simulink model "penddemo"  (R2024a)
settings: Solver=FixedStepAuto  StartTime=0  StopTime=50  FixedStep=0.02  MaxStep=0.02  RelTol=1e-3  AbsTol=1e-6
libraries: slpidlib x1
CloseFcn:
  | set(groot,'ShowHiddenHandles','on');
  | c = get(groot,'Children');
  | close(c);
  | clear c;
  | set(groot,'ShowHiddenHandles','off');
Description:
  | Inverted Pendulum with Animation
  | 
  | This example shows how to model an inverted pendulum.  The animation is created using MATLAB(R) Handle Graphics(R).  The animation block is a masked
  | S-function.  For more information, use the context menu to look under the Animation block's mask
  | and open the S-function for editing.
settings Model: Creator=The MathWorks, Inc.  LastModifiedBy=alexivanov
settings SolverCC: AutoScaleAbsTol=off  AlgebraicLoopSolver=TrustRegion
settings DataIOCC: ExternalInput=[]  InitialState=[]  SaveFormat=Array  SaveOutput=off  SaveTime=off
settings OptimizationCC: BlockReduction=off  BooleanDataType=off  ReuseModelBlockBuffer=off  ExpressionDepthLimit=2147483647  InitFltsAndDblsToZero=on  LifeSpan=inf
settings DebuggingCC: SaveWithParameterizedLinksMsg=none  UnderspecifiedInitializationDetection=Classic  MergeDetectMultiDrivingBlocksExec=none  SignalResolutionControl=TryResolveAllWithWarning  MultiTaskDSMMsg=warning  MultiTaskCondExecSysMsg=none  SigSpecEnsureSampleTimeMsg=none  FcnCallInpInsideContextMsg=warning  UnconnectedInputMsg=warning  UnconnectedOutputMsg=warning  UnconnectedLineMsg=warning  StateNameClashWarn=warning  SubsystemReferenceDiagnosticForUnitTest=warning  SFUnexpectedBacktrackingDiag=warning  SFNoUnconditionalDefaultTransitionDiag=warning  SFExecutionAtInitializationDiag=none  ArithmeticOperatorsInVariantConditions=warning
settings HardwareCC: ProdBitPerPointer=32  ProdBitPerSizeT=32  ProdBitPerPtrDiffT=32  ProdLargestAtomicFloat=None  ProdIntDivRoundTo=Undefined  ProdEndianess=Unspecified  ProdWordSize=32  ProdHWDeviceType=32-bit Generic  TargetUnknown=on
settings ModelReferenceCC: EnableRefExpFcnMdlSchedulingChecks=on  PropagateSignalLabelsOutOfModel=off
settings SFSimCC: SimUseLocalCustomCode=off  CustomCodeUndefinedFunction=UseInterfaceOnly
settings RTWCC: RTWUseLocalCustomCode=off  GPUComputeCapability=3.5
settings CodeAppCC: StateflowObjectComments=on
settings GRTTargetCC: TargetFcnLib=ansi_tfl_tmw.mat  TargetLangStandard=C89/C90 (ANSI)  CombineOutputUpdateFcns=off  GRTInterface=on
settings ConfigComp: CovMetricSettings=dw  CovSaveCumulativeToWorkspaceVar=on  CovSaveSingleToWorkspaceVar=on  CovExternalEMLEnable=off

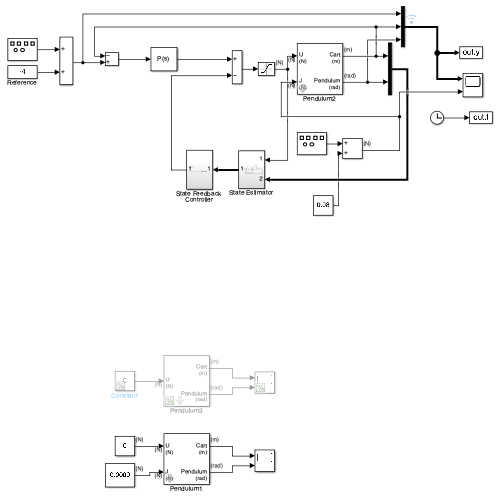
[thumbnail: Simulink's stored preview of the top-level diagram]
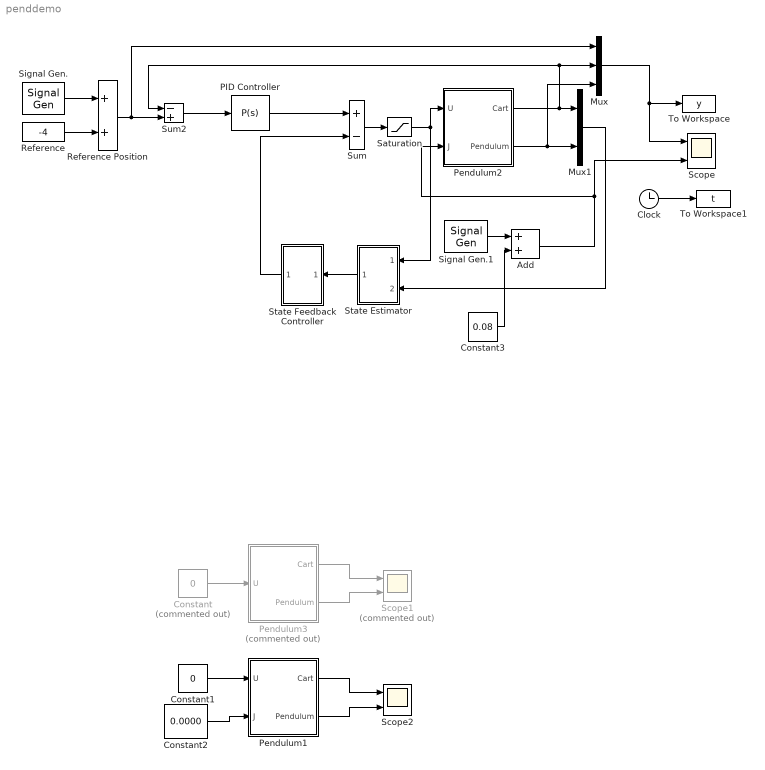
== system penddemo ==
  Add : Sum
  Clock : Clock
  Constant : Constant  Commented=on  Value=0
  Constant1 : Constant  Value=0
  Constant2 : Constant  Value=0.0000
  Constant3 : Constant  Value=0.08
  Mux : Mux  Inputs=3
  Mux1 : Mux  Inputs=2
  "PID Controller " : slpidlib/PID Controller  Controller=P  Form=Parallel  TimeDomain=Continuous-time  UseExternalTs=off  SampleTime=-1  IntegratorMethod=Forward Euler  FilterMethod=Forward Euler  ControllerParametersSource=internal  P=-9.4-4  I=-5  UseKiTs=off  D=0  UseExternalDerivativeSource=off  N=100  UseFilter=on  TunerSelectOption=Transfer Function Based (PID Tuner App)  InitialConditionSource=internal  InitialConditionForIntegrator=0  InitialConditionForFilter=0  DifferentiatorICPrevScaledInput=0  ExternalReset=none  TrackingMode=off  Kt=1  LimitOutput=off  SatLimitsSource=internal  UpperSaturationLimit=inf  LowerSaturationLimit=-inf  LinearizeAsGain=on  AntiWindupMode=none  Kb=1  LimitIntegrator=off  UpperIntegratorSaturationLimit=inf  LowerIntegratorSaturationLimit=-inf  POutMin=[]  POutMax=[]  IOutMin=[]  IOutMax=[]  DOutMin=[]  DOutMax=[]  NOutMin=[]  NOutMax=[]  SumOutMin=[]  SumOutMax=[]  SaturationOutMin=[]  SaturationOutMax=[]  PParamMin=[]  PParamMax=[]  IParamMin=[]  IParamMax=[]  DParamMin=[]  DParamMax=[]  NParamMin=[]  NParamMax=[]  KbParamMin=[]  KbParamMax=[]  KtParamMin=[]  KtParamMax=[]  KbOutMin=[]  KbOutMax=[]  KtOutMin=[]  KtOutMax=[]  IntegratorOutMin=[]  IntegratorOutMax=[]  FilterOutMin=[]  FilterOutMax=[]  SumI1OutMin=[]  SumI1OutMax=[]  SumI2OutMin=[]  SumI2OutMax=[]  SumI3OutMin=[]  SumI3OutMax=[]  SumI4OutMin=[]  SumI4OutMax=[]  SumDOutMin=[]  SumDOutMax=[]  DifferentiatorOutMin=[]  DifferentiatorOutMax=[]  FilterDiffOutCoefMin=[]  FilterDiffOutCoefMax=[]  ReciprocalOutMin=[]  ReciprocalOutMax=[]  SumDenOutMin=[]  SumDenOutMax=[]  SumNumOutMin=[]  SumNumOutMax=[]  DivideOutMin=[]  DivideOutMax=[]  UdiffTsProdOutMin=[]  UdiffTsProdOutMax=[]  NTsProdOutMin=[]  NTsProdOutMax=[]  UintegralTsProdOutMin=[]  UintegralTsProdOutMax=[]  UngainTsProdOutMin=[]  UngainTsProdOutMax=[]  ClampingZeroOutDataTypeStr=Inherit: Inherit via back propagation  ClampingZeroOutMin=[]  ClampingZeroOutMax=[]  FilterDenConstantOutDataTypeStr=Inherit: Inherit via back propagation  FilterDenConstantOutMin=[]  FilterDenConstantOutMax=[]  PCopyOutDataTypeStr=Inherit: Inherit via back propagation  PCopyOutMin=[]  PCopyOutMax=[]  NCopyOutDataTypeStr=Inherit: Inherit via back propagation  NCopyOutMin=[]  NCopyOutMax=[]  IntegratorContinuousStateAttributes=''  IntegratorStateMustResolveToSignalObject=off  IntegratorRTWStateStorageClass=Auto  FilterContinuousStateAttributes=''  FilterStateMustResolveToSignalObject=off  FilterRTWStateStorageClass=Auto  ParallelPVariant=InternalParameters  IdealPVariant=Disabled  IVariant=Disabled  DVariant=Disabled  IntegratorVariant=Disabled  SatVariant=Disabled  AWVariant=Disabled  PCopyVariant=Disabled  TRVariant=Disabled  FdbkBlocksVariant=Forward  IdealPFdbkVariant=Disabled  SatFdbkVariant=Disabled  DerivativeFilterVariant=Disabled  NVariant=Disabled  NCopyVariant=Disabled_SignalSpec  FilterICVariant=Disabled  IntegratorICVariant=Disabled  ExternalResetVariant=Disabled  TRSumVariant=Passthrough  SumFdbkVariant=Disabled  SumVariant=Passthrough_P  TsampFilterVariant=InternalTs  TsampNgainVariant=Passthrough  TsampIntegralVariant=Disabled_SignalSpec  ExternalSaturationOutDataTypeStr=Inherit: Same as second input  DerivativeSourceVariant=Disabled
  Pendulum1 : Subsystem  mask(Inverted Pendulum Dynamics){Mcart=0.455, m=0.21, l=0.61/2, g=9.8}
      mask prompts: Mcart "Mass of cart (kg):"; m "Mass of pendulum (kg):"; l "Distance to pendulum center of mass (m):"; g "Acceleration of gravity (m/s^2):"
      mask help: Masked subsystem containing nonlinear dynamics of inverted pendulum on a cart.
      mask Help: Nonlinear dynamics of inverted pendulum on cart.
  Pendulum2 : Subsystem  mask(Inverted Pendulum Dynamics){Mcart=0.455, m=0.21, l=0.61/2, g=9.8}
      mask prompts: Mcart "Mass of cart (kg):"; m "Mass of pendulum (kg):"; l "Distance to pendulum center of mass (m):"; g "Acceleration of gravity (m/s^2):"
      mask help: Masked subsystem containing nonlinear dynamics of inverted pendulum on a cart.
      mask Help: Nonlinear dynamics of inverted pendulum on cart.
  Pendulum3 : Subsystem  Commented=on  mask(Inverted Pendulum Dynamics){Mcart=0.455, m=0.21, l=0.61/2, g=9.8}
      mask prompts: Mcart "Mass of cart (kg):"; m "Mass of pendulum (kg):"; l "Distance to pendulum center of mass (m):"; g "Acceleration of gravity (m/s^2):"
      mask help: Masked subsystem containing nonlinear dynamics of inverted pendulum on a cart.
      mask Help: Nonlinear dynamics of inverted pendulum on cart.
  Reference : Constant  Value=-4
  Reference Position : Sum  InputSameDT=on  SaturateOnIntegerOverflow=on  OutDataTypeStr=Inherit: Same as first input
  Saturation : Saturate  UpperLimit=100  LowerLimit=-100
  Scope : Scope  NumInputPorts=2
  Scope1 : Scope  Commented=on  NumInputPorts=2
  Scope2 : Scope  NumInputPorts=2
  Signal Gen. : SignalGenerator  WaveForm=square  Frequency=0.2  Units=rad/sec
  Signal Gen.1 : SignalGenerator  WaveForm=square  Amplitude=0.08  Frequency=0.5  Units=rad/sec
  State Estimator : Subsystem
  State Feedback Controller : Subsystem
  Sum : Sum  Inputs=+-  InputSameDT=on  SaturateOnIntegerOverflow=on  OutDataTypeStr=Inherit: Same as first input
  Sum2 : Sum  Inputs=-+  InputSameDT=on  SaturateOnIntegerOverflow=on  OutDataTypeStr=Inherit: Same as first input
  To Workspace : ToWorkspace  VariableName=y  SampleTime=0.1
  To Workspace1 : ToWorkspace  VariableName=t  SampleTime=0.1
  wires:
  Mux/1 -> Scope/1, To Workspace/1
  Pendulum2/2(Pendulum) -> Mux/3, Mux1/2
  Reference Position/1 -> Mux/1, Sum2/2
  Sum2/1 -> "PID Controller "/1
  Sum/1 -> Saturation/1
  Reference/1 -> Reference Position/2
  Signal Gen./1 -> Reference Position/1
  Saturation/1 -> Pendulum2/1(U), State Estimator/1(Input)
  Clock/1 -> To Workspace1/1
  Pendulum2/1(Cart) -> Mux1/1, Sum2/1, Mux/2
  Mux1/1 -> State Estimator/2(Input1)
  "PID Controller "/1 -> Sum/1
  State Estimator/1(Outport) -> State Feedback Controller/1(In1)
  State Feedback Controller/1(Out1) -> Sum/2
  Constant/1 -> Pendulum3/1(U)
  Pendulum3/1(Cart) -> Scope1/1
  Pendulum3/2(Pendulum) -> Scope1/2
  Pendulum1/1(Cart) -> Scope2/1
  Pendulum1/2(Pendulum) -> Scope2/2
  Constant1/1 -> Pendulum1/1(U)
  Constant2/1 -> Pendulum1/2(J)
  Add/1 -> Scope/2, Pendulum2/2(J)
  Signal Gen.1/1 -> Add/1
  Constant3/1 -> Add/2

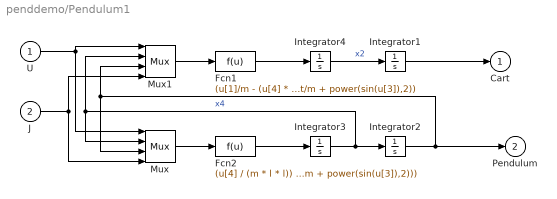
== system penddemo/Pendulum1 ==
  U : Inport  Unit=N
  J : Inport  Port=2  Unit=N
  Fcn1 : Fcn  Expr=(u[1]/m - (u[4] * cos(u[3]) / (m * l)) - g*sin(u[3])*cos(u[3]) + l*power(u[2],2)*sin(u[3]))/(Mcart/m + power(sin(u[3]),2))
  Fcn2 : Fcn  Expr=(u[4] / (m * l * l)) + (-u[1]*cos(u[3])/m + (u[4] * power(cos(u[4]), 2) / (l * m)) + (Mcart+m)*g*sin(u[3])/m - l*power(u[2],2)*sin(u[3])*cos(u[3]))/(l*(Mcart/m + power(sin(u[3]),2)))
  Integrator{1..4} (4 alike) : Integrator
  Mux : Mux
  Mux1 : Mux
  Cart : Outport  Unit=m  InitialOutput=0  VectorParamsAs1DForOutWhenUnconnected=off
  Pendulum : Outport  Port=2  Unit=rad  InitialOutput=0  VectorParamsAs1DForOutWhenUnconnected=off
  wires:
  Integrator1/1 -> Cart/1
  Fcn2/1 -> Integrator3/1
  Mux/1 -> Fcn2/1
  Mux1/1 -> Fcn1/1
  Fcn1/1 -> Integrator4/1
  Integrator4/1 -> Integrator1/1  "x2"
  U/1 -> Mux1/1, Mux/1
  Integrator3/1 -> Integrator2/1, Mux1/2, Mux/2  "x4"
  Integrator2/1 -> Pendulum/1, Mux1/3, Mux/3
  J/1 -> Mux/4, Mux1/4

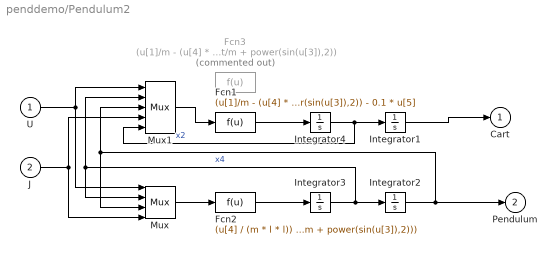
== system penddemo/Pendulum2 ==
  U : Inport  Unit=N
  J : Inport  Port=2  Unit=N
  Fcn1 : Fcn  Expr=(u[1]/m - (u[4] * cos(u[3]) / (m * l)) - g*sin(u[3])*cos(u[3]) + l*power(u[2],2)*sin(u[3]))/(Mcart/m + power(sin(u[3]),2)) - 0.1 * u[5]
  Fcn2 : Fcn  Expr=(u[4] / (m * l * l)) + (-u[1]*cos(u[3])/m + (u[4] * power(cos(u[4]), 2) / (l * m)) + (Mcart+m)*g*sin(u[3])/m - l*power(u[2],2)*sin(u[3])*cos(u[3]))/(l*(Mcart/m + power(sin(u[3]),2)))
  Fcn3 : Fcn  Commented=on  Expr=(u[1]/m - (u[4] * cos(u[3]) / (m * l)) - g*sin(u[3])*cos(u[3]) + l*power(u[2],2)*sin(u[3]))/(Mcart/m + power(sin(u[3]),2))
  Integrator{1..4} (4 alike) : Integrator
  Mux : Mux
  Mux1 : Mux  Inputs=5
  Cart : Outport  Unit=m  InitialOutput=0  VectorParamsAs1DForOutWhenUnconnected=off
  Pendulum : Outport  Port=2  Unit=rad  InitialOutput=0  VectorParamsAs1DForOutWhenUnconnected=off
  wires:
  Integrator1/1 -> Cart/1
  Fcn2/1 -> Integrator3/1
  Mux/1 -> Fcn2/1
  Mux1/1 -> Fcn1/1
  Fcn1/1 -> Integrator4/1
  Integrator4/1 -> Integrator1/1, Mux1/5  "x2"
  U/1 -> Mux1/1, Mux/1
  Integrator3/1 -> Integrator2/1, Mux1/2, Mux/2  "x4"
  Integrator2/1 -> Pendulum/1, Mux1/3, Mux/3
  J/1 -> Mux/4, Mux1/4

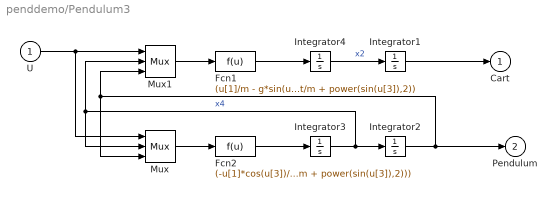
== system penddemo/Pendulum3 ==
  U : Inport  Unit=N
  Fcn1 : Fcn  Expr=(u[1]/m - g*sin(u[3])*cos(u[3]) + l*power(u[2],2)*sin(u[3]))/(Mcart/m + power(sin(u[3]),2))
  Fcn2 : Fcn  Expr=(-u[1]*cos(u[3])/m + (Mcart+m)*g*sin(u[3])/m - l*power(u[2],2)*sin(u[3])*cos(u[3]))/(l*(Mcart/m + power(sin(u[3]),2)))
  Integrator1 : Integrator
  Integrator2 : Integrator  InitialCondition=-pi/2
  Integrator3 : Integrator
  Integrator4 : Integrator
  Mux : Mux  Inputs=3
  Mux1 : Mux  Inputs=3
  Cart : Outport  Unit=m  InitialOutput=0  VectorParamsAs1DForOutWhenUnconnected=off
  Pendulum : Outport  Port=2  Unit=rad  InitialOutput=0  VectorParamsAs1DForOutWhenUnconnected=off
  wires:
  Integrator1/1 -> Cart/1
  Fcn2/1 -> Integrator3/1
  Mux/1 -> Fcn2/1
  Mux1/1 -> Fcn1/1
  Fcn1/1 -> Integrator4/1
  Integrator4/1 -> Integrator1/1  "x2"
  U/1 -> Mux1/1, Mux/1
  Integrator3/1 -> Integrator2/1, Mux1/2, Mux/2  "x4"
  Integrator2/1 -> Pendulum/1, Mux1/3, Mux/3

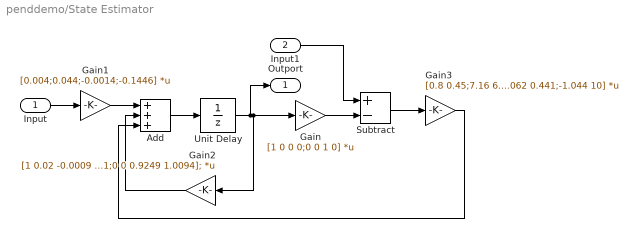
== system penddemo/State Estimator ==
  Input : Inport
  Input1 : Inport  Port=2
  Add : Sum  Inputs=+++
  Gain : Gain  Gain=[1 0 0 0;0 0 1 0]  Multiplication=Matrix(K*u)
  Gain1 : Gain  Gain=[0.004;0.044;-0.0014;-0.1446]  Multiplication=Matrix(K*u)
  Gain2 : Gain  Gain=[1 0.02 -0.0009 0;0 1 -0.0907 -0.0009;0 0 1.0094 0.0201;0 0 0.9249 1.0094];  Multiplication=Matrix(K*u)
  Gain3 : Gain  Gain=[0.8 0.45;7.16 6.28;-0.062 0.441;-1.044 10]  Multiplication=Matrix(K*u)
  Subtract : Sum  Inputs=+-
  Unit Delay : UnitDelay  InitialCondition=zeros(4,1)  SampleTime=-1  HasFrameUpgradeWarning=on
  Outport : Outport
  wires:
  Unit Delay/1 -> Gain/1, Gain2/1, Outport/1
  Gain1/1 -> Add/1
  Add/1 -> Unit Delay/1
  Subtract/1 -> Gain3/1
  Input/1 -> Gain1/1
  Gain2/1 -> Add/2
  Gain/1 -> Subtract/2
  Input1/1 -> Subtract/1
  Gain3/1 -> Add/3

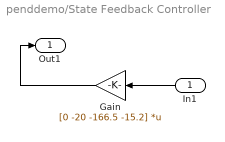
== system penddemo/State Feedback Controller ==
  In1 : Inport
  Gain : Gain  Gain=[0 -20 -166.5 -15.2]  Multiplication=Matrix(K*u)
  Out1 : Outport
  wires:
  Gain/1 -> Out1/1
  In1/1 -> Gain/1
